simulink model "bank_block_example"  (Simulink 8.6)
settings: Solver=FixedStepDiscrete  SolverMode=SingleTasking  StartTime=0.0  StopTime=120.0  RelTol=1e-3
libraries: moneylib x3
settings Model: Creator=gcampa  LastModifiedBy=gcampa
settings DataIOCC: LimitDataPoints=off  SaveFormat=Dataset  SignalLoggingSaveFormat=Dataset  ReturnWorkspaceOutputs=on
settings OptimizationCC: ExpressionDepthLimit=128
settings DebuggingCC: UnderspecifiedInitializationDetection=Simplified  MergeDetectMultiDrivingBlocksExec=error  SolverPrmCheckMsg=none  FcnCallInpInsideContextMsg=EnableAllAsError  AllowSymbolicDim=on  StateNameClashWarn=none  SFUnexpectedBacktrackingDiag=error  SFNoUnconditionalDefaultTransitionDiag=error
settings HardwareCC: ProdBitPerPointer=64  ProdLargestAtomicFloat=Float  ProdIntDivRoundTo=Zero  ProdEndianess=LittleEndian  ProdWordSize=64  ProdHWDeviceType=Intel->x86-64 (Windows64)
settings ModelReferenceCC: PropagateSignalLabelsOutOfModel=on
settings SFSimCC: SimUseLocalCustomCode=on
settings RTWCC: RTWUseLocalCustomCode=on
settings GRTTargetCC: TargetLangStandard=C99 (ISO)  GeneratePreprocessorConditionals=Use local settings  CombineOutputUpdateFcns=on  GRTInterface=off
settings ConfigComp: CovMetricSettings=dwe  CovSaveCumulativeToWorkspaceVar=off  CovSaveSingleToWorkspaceVar=off  CovExternalEMLEnable=on

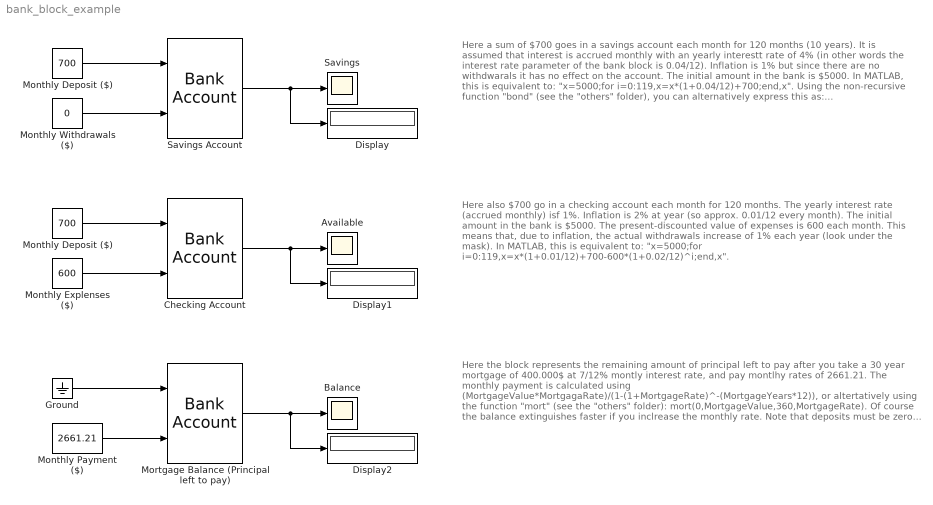
== system bank_block_example ==
  note: Here a sum of $700 goes in a savings account each month for 120 months (10 years).
      | It is assumed that interest is accrued monthly with an yearly interestt rate of 4% (in other words the interest rate parameter of the bank block is 0.04/12). Inflation is 1% but since there are no withdwarals it has no effect on the account. The initial amount in the bank is $5000.
      |
      | In MATLAB, this is equivalent to: "x=5000;for i=0:119,x=x*(1+0.04/12)+700;end,x".
      | Using the non-recursive function "bond" (see the "others" folder), you can alternatively express this as: "bond(5000,-700,-120,0.04/12)". Look under the mask for more insight.
      | Also, bank=ss(1+0.04/12,1,1,0,1);y=lsim(bank,700*ones(1,121),0:120,5000);y(end)
      | >> y=lsim(bank,700*ones(1,121),0:120,5000);y(end)
  note: Here also $700 go in a checking account each month for 120 months. The yearly interest rate (accrued monthly) isf 1%. Inflation is 2% at year (so approx. 0.01/12 every month). The initial amount in the bank is $5000.
      | The present-discounted value of expenses is 600 each month. This means that, due to inflation, the actual withdrawals increase of 1% each year (look under the mask).
      |
      | In MATLAB, this is equivalent to:
      | "x=5000;for i=0:119,x=x*(1+0.01/12)+700-600*(1+0.02/12)^i;end,x".
  note: Here the block represents the remaining amount of principal left to pay after you take a 30 year mortgage of 400.000$ at 7/12% montly interest rate, and pay montlhy rates of 2661.21. The monthly payment is calculated using (MortgageValue*MortgagaRate)/(1-(1+MortgageRate)^-(MortgageYears*12)), or altertatively using the function "mort" (see the "others" folder): mort(0,MortgageValue,360,MortgageRate). Of course the balance extinguishes faster if you inclrease the monthly rate. Note that deposits must be zero (you don't add to the borrowed balance) and inflation must be zero (unless you plan to increase your payments exponentially with time.
      |
      | In MATLAB, this is equivalent to
      | "x=400000;for i=0:119,x=x*(1+0.07/12)-2661.21;end,x".
  Available : Scope
  Balance : Scope
  Checking Account : moneylib/Bank Account  i=0.01/12  j=0.02/12  x0=5000
  Display : Display
      settings: Format=bank
  Display1 : Display
      settings: Format=bank
  Display2 : Display
      settings: Format=bank
  Ground : Ground
  Monthly Deposit ($) : Constant  Value=700
  "Monthly Deposit ($) " : Constant  Value=700
  Monthly Explenses ($) : Constant  Value=600
  Monthly Payment ($) : Constant  Value=2661.21
  Monthly Withdrawals ($) : Constant  Value=0
  Mortgage Balance (Principal left to pay) : moneylib/Bank Account  i=0.07/12  j=0  x0=400000
  Savings : Scope
  Savings Account : moneylib/Bank Account  i=0.04/12  j=0.01/12  x0=5000
  wires:
  Savings Account/1 -> Display/1, Savings/1
  Monthly Deposit ($)/1 -> Savings Account/1
  Monthly Withdrawals ($)/1 -> Savings Account/2
  Monthly Explenses ($)/1 -> Checking Account/2
  Checking Account/1 -> Display1/1, Available/1
  "Monthly Deposit ($) "/1 -> Checking Account/1
  Monthly Payment ($)/1 -> Mortgage Balance (Principal left to pay)/2
  Mortgage Balance (Principal left to pay)/1 -> Display2/1, Balance/1
  Ground/1 -> Mortgage Balance (Principal left to pay)/1
